simulink model "lander12_11no2"  (R2018a)
settings: Solver=VariableStepAuto  StartTime=0.0  StopTime=150  RelTol=1e-3
undefined symbols (not defined in the file or in its folder): myu, R
libraries: simulink_extras x2
settings Model: Creator=hp731  LastModifiedBy=hp731

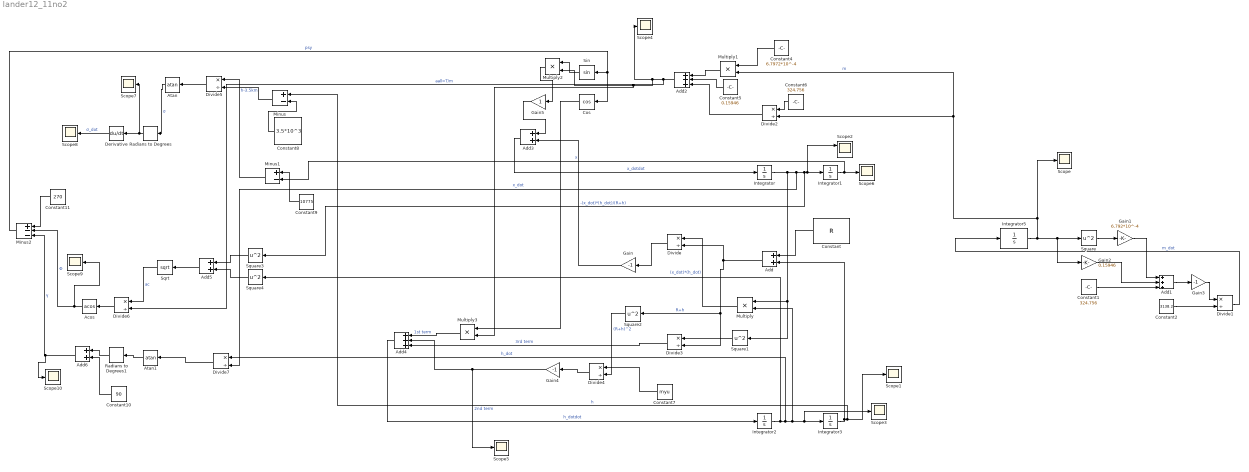
== system lander12_11no2 ==
  Acos : Trigonometry  Operator=acos
  Add{,3,5..6} (4 alike) : Sum
  Add1 : Sum  Inputs=+++
  Add2 : Sum  Inputs=+++
  Add4 : Sum  Inputs=+++
  Atan : Trigonometry  Operator=atan
  Atan1 : Trigonometry  Operator=atan
  Constant : Constant  Value=R
  Constant1 : Constant  Value=324.756
  Constant10 : Constant  Value=90
  Constant11 : Constant  Value=270
  Constant2 : Constant  Value=3138.2
  Constant4 : Constant  Value=6.7972*10^-4
  Constant5 : Constant  Value=0.15946
  Constant6 : Constant  Value=324.756
  Constant7 : Constant  Value=myu
  Constant8 : Constant  Value=3.5*10^3
  Constant9 : Constant  Value=10775
  Cos : Trigonometry  Operator=cos
  Derivative : Derivative
  Divide{,1..3,5..7} (7 alike) : Product  Inputs=*/
  Divide4 : Product  Inputs=*/  SaturateOnIntegerOverflow=on  RndMeth=Zero
  Gain : Gain  Gain=-1
  Gain1 : Gain  Gain=6.792*10^-4
  Gain2 : Gain  Gain=0.15946
  Gain3 : Gain  Gain=-1
  Gain4 : Gain  Gain=-1
  Gain5 : Gain
  Integrator : Integrator  InitialCondition=186.55
  Integrator1 : Integrator
  Integrator2 : Integrator  InitialCondition=-97.02
  Integrator3 : Integrator  InitialCondition=14275
  Integrator5 : Integrator  InitialCondition=165.33
  Minus : Sum  Inputs=+-
  Minus1 : Sum  Inputs=+-
  Minus2 : Sum  Inputs=+--
  Multiply{,1..3} (4 alike) : Product
  Radians to Degrees : simulink_extras/Transformations/Radians to Degrees
  Radians to Degrees1 : simulink_extras/Transformations/Radians to Degrees
  Scope{,1,3..10} (10 alike) : Scope
  Scope2 : Scope  NumInputPorts=2
  Sin : Trigonometry
  Sqrt : Sqrt  SaturateOnIntegerOverflow=on
  Square{,1..4} (5 alike) : Math  Operator=square  SaturateOnIntegerOverflow=on
  wires:
  Add3/1 -> Integrator/1  "x_dotdot"
  Integrator/1 -> Square1/1, Multiply/1, Divide7/2, Square3/1, Scope2/1, Integrator1/1  "x_dot"
  Integrator2/1 -> Square4/1, Divide7/1, Multiply/2, Scope3/1, Integrator3/1  "h_dot"
  Integrator3/1 -> Minus/1, Scope1/1, Add/2  "h"
  Add4/1 -> Integrator2/1  "h_dotdot"
  Constant/1 -> Add/1
  Add/1 -> Square2/1, Divide3/2, Divide/2  "R+h"
  Multiply/1 -> Divide/1  "(x_dot)*(h_dot)"
  Divide/1 -> Gain/1
  Gain/1 -> Add3/2  "-(x_dot)*(h_dot)/(R+h)"
  Integrator5/1 -> Divide2/2, Multiply1/2, Scope/1, Gain2/1, Square/1  "m"
  Divide1/1 -> Integrator5/1  "m_dot"
  Square/1 -> Gain1/1
  Gain1/1 -> Add1/1
  Gain2/1 -> Add1/2
  Constant1/1 -> Add1/3
  Add1/1 -> Gain3/1
  Gain3/1 -> Divide1/1
  Constant2/1 -> Divide1/2
  Constant4/1 -> Multiply1/1
  Multiply1/1 -> Add2/1
  Constant5/1 -> Add2/2
  Constant6/1 -> Divide2/1
  Divide2/1 -> Add2/3
  Add2/1 -> Divide6/2, Scope4/1, Multiply3/2, Multiply2/2  "aall=T/m"
  Sin/1 -> Multiply2/1
  Multiply2/1 -> Gain5/1
  Square1/1 -> Divide3/1
  Constant7/1 -> Divide4/1
  Square2/1 -> Divide4/2  "(R+h)^2"
  Divide4/1 -> Gain4/1
  Gain4/1 -> Scope5/1, Add4/2  "2nd term"
  Divide3/1 -> Add4/3  "3rd term"
  Cos/1 -> Multiply3/1
  Multiply3/1 -> Add4/1  "1st term"
  Gain5/1 -> Add3/1
  Integrator1/1 -> Minus1/2, Scope6/1  "x"
  Constant8/1 -> Minus/2
  Minus/1 -> Divide5/2  "h-3.5km"
  Divide5/1 -> Atan/1
  Atan/1 -> Radians to Degrees/1  "σ"
  Radians to Degrees/1 -> Derivative/1, Scope7/1
  Constant9/1 -> Minus1/1
  Minus1/1 -> Divide5/1
  Derivative/1 -> Scope8/1  "σ_dot"
  Square3/1 -> Add5/1
  Square4/1 -> Add5/2
  Add5/1 -> Sqrt/1
  Sqrt/1 -> Divide6/1  "ac"
  Divide6/1 -> Acos/1
  Acos/1 -> Scope9/1, Minus2/2  "Φ"
  Divide7/1 -> Atan1/1
  Atan1/1 -> Radians to Degrees1/1
  Radians to Degrees1/1 -> Add6/1
  Constant10/1 -> Add6/2
  Add6/1 -> Scope10/1, Minus2/3  "γ"
  Constant11/1 -> Minus2/1
  Minus2/1 -> Cos/1, Sin/1  "psy"
